simulink model "tqdtqr_rebuild_V3"  (R2021b)
settings: Solver=VariableStepAuto  StartTime=0.0  StopTime=10.0  RelTol=1e-3
undefined symbols (not defined in the file): ATQD_AfterTqMinGain_X_Deg, ATQD_APSCreepBaseTqD_X_kph, ATQD_APSCreepBaseTqD_Y_Deg, ATQD_APSCreepBaseTqR_X_kph, ATQD_APSCreepBaseTqR_Y_Deg, ATQD_APSCreepIterm_X_kph, ATQD_APSCreepIterm_Y_kph, ATQD_APSCreepPterm_X_kph, ATQD_APSCreepPterm_Y_kph, ATQD_APSDecReq_X_kph, ATQD_APSDecReq_Y_mps2, ATQD_APSDecReqCMD_X_kph, ATQD_APSDecReqTs_X_pct, ATQD_APSDecTimeGain_X_Deg, ATQD_APSDecTimeGain_Y_s, ATQD_APSReqLowSpd_X_Deg, ATQD_AutoHoldReleaseBPS_X_Deg, ATQD_AWDLoadTrqnsGain_X_kg, ATQD_AWDLoadTrqnsGain_Y_pct, ATQD_BOSEnBPSPosn_X_kph, ATQD_BOSMap_X_rpm, ATQD_BOSMap_Y_pct, ATQD_CreepBaseTqD_X_kph, ATQD_CreepBaseTqD_Y_Deg, ATQD_CreepBaseTqR_X_kph, ATQD_CreepBaseTqR_Y_Deg, ATQD_CreepBPSDisPosn_X_Deg, ATQD_CreepBPSDisPosnR_X_Deg, ATQD_CreepBPSEnPosn_X_Deg, ATQD_CreepBPSEnPosnR_X_Deg, ATQD_CreepDeltaTq_X_kph, ATQD_CreepIterm_X_kph, ATQD_CreepIterm_Y_kph, ATQD_CreepItermMaxLimit_X_pct, ATQD_CreepPreloadTime_X_kph, ATQD_CreepPreloadTq_X_kph, ATQD_CreepPreloadTq_Y_s, ATQD_CreepProtTq_X_Deg, ATQD_CreepPterm_X_kph, ATQD_CreepPterm_Y_kph, ATQD_CreepRrTqSpRat_X_rpm, ATQD_CreepRrTqSpRat_Y_Nm, ATQD_CreepTargetSpdD_X_pct, ATQD_CreepTargetSpdR_X_pct, ATQD_CreepUpLimitTq_X_rpm, ATQD_DecIneOPDHoldEnDelay_X_Deg, ATQD_DecIneOPDHoldEnDelay_Y_bar, ATQD_ECOTqMapD_X_rpm, ATQD_ECOTqMapD_Y_pct, ATQD_EMTqMapD_X_rpm, ATQD_EMTqMapD_Y_pct, ATQD_EOPDTqMapDCon_X_rpm, ATQD_EOPDTqMapDCon_Y_Deg, ATQD_EstInitVehWeight_X_c, ATQD_FAfterTqCMDGain_X_rpm, ATQD_FAfterTqCMDGain_Y_pct, ATQD_ForceLowSpd_X_Deg, ATQD_ForcePLimitSpd_X_Deg, ATQD_FrLossMAPLowV_X_rpm, ATQD_FrLossMAPLowV_Y_Nm ... (+949)
libraries: simulink x235, hcu_lib x208, tqr x63, tqd x6
(part 18 of 37)

== system tqdtqr_rebuild_V3/Input_Convert/Main function/DriverWhlTqDem function/PedalMapWhlTq ==
  note: Slide rate/SAS/YawRate regen torque
  note: According conditons use different torque, upper and lower limits
  note: Road slope
  note: Pedal map final torque
  note: Cancel ACC condition
  note: ACC shut off
  BSCPIn_outputs : Inport
  BSignalConvert_outputs : Inport  Port=2
  VTQD_PedAccTqEn_flg : Inport  Port=3
  VTQD_PedalTqCal_Nm : Inport  Port=4
  VTQD_PedalMapWhlTqMerge_Nm : Inport  Port=5
  BMain_outputs : Inport  Port=6
  BFunction_outputs : Inport  Port=7
  AND{,1..4,6} (6 alike) : Logic  AllPortsSameDT=off  OutDataTypeStr=boolean
  AND5 : Logic  Inputs=3  AllPortsSameDT=off  OutDataTypeStr=boolean
  AND7 : Logic  Operator=OR  AllPortsSameDT=off  OutDataTypeStr=boolean
  Abs{,1..3} (4 alike) : Abs
  Add : Sum  Inputs=+-
  Add1 : Sum
  Add13 : Sum  Inputs=+-
  Add2 : Sum
  Add3 : Sum
  Add4 : Sum  Inputs=+-
  Bus Selector : BusSelector  OutputSignals=VVMC_EstSlope_Deg,VINP_RrPTCSActive_flg,VINP_FrPTCSActive_flg,VINP_ADASACCSta_enum,VTQD_LowIdleAccPedal_flg,VVMC_ADASActive_flg,VVMC_ActMaxSlideRate_pct,VVMC_LongAcc_Gps,VINP_SASAngle_Deg,VINP_YawRate_degps,VVMC_ActStESCYaw_Dps,VINP_BrkPedalPos_pct,VTQD_ActAPSPosn_pct,VVMC_ADASWhlTqReq_Nm,VINP_HSAActive_flg
  Bus Selector1 : BusSelector  OutputSignals=VTQD_BrkSwSta_flg,VTQD_RollRegenDisable_flg,VTQD_TqTargetShaftSpd_rpm,VTQD_VehActSpd_kph
  Bus Selector2 : BusSelector  OutputSignals=VTQD_OPDHoldEnRel_flg
  Bus Selector3 : BusSelector  OutputSignals=VTQR_NoABSREDUWhlTqReq_Nm,VTQR_NoABSFEDUWhlTqReq_Nm
  Constant1 : Constant  Value=KTQD_RgnEnLatchSpd_kph
  Constant10 : Constant  Value=KTQD_ClimbMin_rpm
  Constant11 : Constant  Value=KTQD_PedalMapRDCUpLim_Nm
  Constant12 : Constant  Value=KTQD_PedalMapRDCLowLim_Nm
  Constant13 : Constant  Value=KTQD_GRADE_Deg_ovrdval
  Constant14 : Constant  Value=KTQD_PedalMapRDCUpLim_Nm
  Constant15 : Constant  Value=KTQD_TargetSlideRate_pct
  Constant16 : Constant  Value=KTQD_SlideRateDevUpLim_pct
  Constant17 : Constant  Value=KTQD_SlideRateDevLowLim_pct
  Constant18 : Constant  Value=KTQD_PedalMapRDCLowLim_Nm
  Constant19 : Constant  Value=KTQD_SlideRegEnLimitTq_Nm
  Constant20 : Constant  Value=KTQD_SlideRegEnLimitTq_Nm
  Constant21 : Constant  Value=KTQD_OrigPedTqLowLimSW_flg
  Constant22 : Constant  Value=KTQD_PedalMapRDCLowLim_Nm
  Constant23 : Constant  Value=KTQD_SlideRegenLowLim_Nm
  Constant24 : Constant  Value=KTQD_RgnEnLatchBrkPos_pct
  Constant25 : Constant  Value=ENUM_ADASACCSTA_SHUTOFF
  Constant26 : Constant  Value=KTQD_RgnEnLatchBrkPos_pct
  Constant27 : Constant  Value=KTQD_RgnEnLatchSlope_Deg
  Constant28 : Constant  Value=ZERO_FLOAT
  Constant29 : Constant  Value=ENUM_ADASACCSTA_STANDBY
  Constant30 : Constant  Value=ENUM_ADASACCSTA_OFF
  Constant31 : Constant  Value=KTQD_ACCOvrdCancelResPedTq_pct
  Constant32 : Constant  Value=KTQD_ACCOvrdCancelTqCtrl_flg
  Constant33 : Constant  Value=KVMC_ACCOvrdTestSW_flg
  Constant4 : Constant  Value=KTQD_GRADE_Deg_ovrdflg
  Constant5 : Constant  Value=KTQD_PedalMapClimbLowLim_Nm
  Constant69 : Constant  Value=KTQD_ACCOvrdCancelPedTqRat_Nm
  Constant72 : Constant  Value=ENUM_ADASACCSTA_OVERRIDE
  Delay : Delay  DelayLength=1
  Delay1 : Delay  DelayLength=1
  Delay2 : Delay  DelayLength=1
  Delay3 : Delay  DelayLength=1  InitialCondition=single(0)
      settings: AttributesFormatString=%<InitialCondition>
  Delay4 : Delay  DelayLength=1  InitialCondition=single(0)
      settings: AttributesFormatString=%<InitialCondition>
  Detect Decrease : simulink/Logic and Bit Operations/Detect Decrease  vinit=0.0  OutDataTypeStr=boolean
  Detect Increase : simulink/Logic and Bit Operations/Detect Increase  vinit=0.0  OutDataTypeStr=boolean
  Detect Increase1 : simulink/Logic and Bit Operations/Detect Increase  vinit=0.0  OutDataTypeStr=boolean
  Divide7 : Product  Inputs=**
  Equal : RelationalOperator  Operator===  OutDataTypeStr=boolean  RndMeth=Simplest
  Logical Operator2 : Logic  Operator=OR  Inputs=3  AllPortsSameDT=off  OutDataTypeStr=boolean
  Logical Operator3 : Logic  Operator=OR  AllPortsSameDT=off  OutDataTypeStr=boolean
  MTQD_OrigPedTqLowLim_Z_Nm : Lookup_n-D  BreakpointsForDimension1=ATQD_OrigPedTqLowLim_Y_pct  BreakpointsForDimension2=ATQD_OrigPedTqLowLim_X_Deg  Table=MTQD_OrigPedTqLowLim_Z_Nm  ExtrapMethod=Clip  InternalRulePriority=Speed  RndMeth=Simplest  InputSameDT=on
      settings: InputPortMap=u0,u1
  MTQD_PedalMapClimbUpLim_Z_Nm : Lookup_n-D  BreakpointsForDimension1=ATQD_PedalMapClimbUpLim_Y_Deg  BreakpointsForDimension2=ATQD_PedalMapClimbUpLim_X_rpm  Table=MTQD_PedalMapClimbUpLim_Z_Nm  ExtrapMethod=Clip  InternalRulePriority=Speed  RndMeth=Simplest  InputSameDT=on
      settings: InputPortMap=u0,u1
  "MTQD_SlideRegenTqGain_Z_Nm " : Lookup_n-D  BreakpointsForDimension1=ATQD_SlideRegenTqGain_Y_pct  BreakpointsForDimension2=ATQD_SlideRegenTqGain_X_Gps  Table=MTQD_SlideRegenTqGain_Z_Nm  ExtrapMethod=Clip  InternalRulePriority=Speed  RndMeth=Simplest  InputSameDT=on
      settings: InputPortMap=u0,u1
  MTQD_YawTqLowLim_Y_Nm : Lookup_n-D  NumberOfTableDimensions=1  BreakpointsForDimension1=ATQD_YawTqLowLim_X_degps  Table=MTQD_YawTqLowLim_Y_Nm  ExtrapMethod=Clip  InternalRulePriority=Speed  RndMeth=Simplest  InputSameDT=on
  Max{,1..3} (4 alike) : MinMax  Function=max  Inputs=2
  Min : MinMax  Inputs=2
  NOT : Logic  Operator=NOT  AllPortsSameDT=off  OutDataTypeStr=boolean
  NOT1 : Logic  Operator=NOT  AllPortsSameDT=off  OutDataTypeStr=boolean
  OR{,1..3} (4 alike) : Logic  Operator=OR  AllPortsSameDT=off  OutDataTypeStr=boolean
  Relational Operator{,1,3,6,9,12} (6 alike) : RelationalOperator  Operator=<=  OutDataTypeStr=boolean  RndMeth=Simplest
  Relational Operator10 : RelationalOperator  OutDataTypeStr=boolean  RndMeth=Simplest
  Relational Operator11 : RelationalOperator  OutDataTypeStr=boolean  RndMeth=Simplest
  Relational Operator2 : RelationalOperator  Operator=>  OutDataTypeStr=boolean  RndMeth=Simplest
  Relational Operator4 : RelationalOperator  Operator===  OutDataTypeStr=boolean  RndMeth=Simplest
  Relational Operator5 : RelationalOperator  Operator=>  OutDataTypeStr=boolean  RndMeth=Simplest
  Relational Operator7 : RelationalOperator  Operator===  OutDataTypeStr=boolean  RndMeth=Simplest
  Relational Operator8 : RelationalOperator  Operator===  OutDataTypeStr=boolean  RndMeth=Simplest
  SR_Latch{,1..4} (5 alike) : hcu_lib/Basic_Blocks/SR_Latch
  Saturation Dynamic{,1..4} (5 alike) : simulink/Discontinuities/Saturation Dynamic  OutMin=[]  OutMax=[]  OutDataTypeStr=Inherit: Same as second input  OutDataType=fixdt(1, 16)  OutScaling=2^-10  DoSatur=off
  Switch{3..8,10..12} (9 alike) : Switch  Criteria=u2 ~= 0
      Switch10 settings: AttributesFormatString=%<Criteria>
      Switch11 settings: AttributesFormatString=%<Criteria>
      Switch12 settings: AttributesFormatString=%<Criteria>
      Switch3 settings: AttributesFormatString=%<Criteria>
      Switch4 settings: AttributesFormatString=%<Criteria>
      Switch6 settings: AttributesFormatString=%<Criteria>
      Switch7 settings: AttributesFormatString=%<Criteria>
      Switch8 settings: AttributesFormatString=%<Criteria>
  Switch9 : Switch  Criteria=u2 > Threshold
  Triggered Subsystem : Subsystem  TreatAsAtomicUnit=on
  Unit Delay : UnitDelay  SampleTime=-1  HasFrameUpgradeWarning=on
  VTQD_PedalMapWhlTq_Nm : Outport
  VTQD_PreDecTqLowLim_Nm : Outport  Port=2
  VTQD_RegenTqLimitEn_flg : Outport  Port=3
  VTQD_SlideRegenLimTq_Nm : Outport  Port=4
  wires:
  [VTQD_RollRegenDisableReq_flg] -> Detect Decrease/1
  Relational Operator5/1 -> AND4/1
  [VTQR_NoABSFEDUWhlTqReq_Nm] -> Delay4/1
  [VTQD_BrkSwSta_flg] -> OR/2
  [VTQD_ACCCancelMemTq_Nm] -> Relational Operator11/2
  [VINP_BrkPedalPos_pct] -> Relational Operator5/1
  Constant5/1 -> Saturation Dynamic/3
  SR_Latch2/1 -> Switch9/2, Switch10/2  "VTQD_BrkRgnLatchEn_flg"
  [VTQD_LowIdleAccPedal_flg] -> NOT1/1
  Relational Operator3/1 -> AND7/1
  Switch9/1 -> [VTQD_BrkRgnLatchTqLim_Nm]  "VTQD_BrkRgnLatchTqLim_Nm"
  Delay1/1 -> OR1/1
  Constant24/1 -> Relational Operator3/2
  Constant69/1 -> Divide7/2
  [VTQD_ACCCancelMemTq_Nm] -> Max2/2
  Triggered Subsystem/2(Out2) -> [VTQD_ACCCancelMemPosn_pct]  "VTQD_ACCCancelMemPosn_pct"
  AND7/1 -> SR_Latch2/2
  Relational Operator10/1 -> Switch11/2
  Max2/1 -> Switch11/1
  AND5/1 -> SR_Latch4/1, Detect Increase1/1
  Relational Operator11/1 -> OR3/2
  Add3/1 -> Max3/2
  [VTQD_ActAPSPosn_pct] -> Relational Operator10/1
  Constant21/1 -> AND2/2
  Constant28/1 -> Min/2
  [VTQD_ACCCancelMemTq_Nm] -> Add3/1
  [VVMC_EstSlope_Deg] -> Switch5/3
  [VTQD_PedalTqCal_Nm] -> Switch12/1
  Min/1 -> Switch9/1
  [VVMC_EstSlope_Deg] -> Relational Operator6/1
  Relational Operator6/1 -> AND4/2
  [VINP_BrkPedalPos_pct] -> Relational Operator3/1
  Switch11/1 -> Switch7/1
  SR_Latch4/1 -> [VTQD_ACCCancelDet_flg]  "VTQD_ACCCancelDet_flg"
  OR2/1 -> AND5/2
  [VTQD_VehActSpd_kph] -> Relational Operator12/1
  Abs3/1 -> MTQD_OrigPedTqLowLim_Z_Nm/2
  Triggered Subsystem/1(Out1) -> [VTQD_ACCCancelMemTq_Nm]  "VTQD_ACCCancelMemTq_Nm"
  [VINP_YawRate_degps] -> Abs2/1
  Relational Operator9/1 -> OR3/1
  [VVMC_ActStESCYaw_degps] -> Add4/2
  Relational Operator8/1 -> OR2/2
  [VTQD_ActAPSPosn_pct] -> Add13/1
  AND2/1 -> Switch8/2
  [VVMC_LastADASWhlTqReq_Nm] -> Triggered Subsystem/1(in1)
  [VTQD_ActPedalMapWhlTq_Nm] -> Max3/1
  [VTQD_ActPedalMapWhlTq_Nm] -> Max2/1
  [VTQD_SlideTqLowLim_Nm] -> Switch9/3
  [VTQD_ActPedalMapWhlTq_Nm] -> Switch7/3
  [VTQD_OrigPedalMapWhlTq_Nm] -> Relational Operator2/1
  Switch4/1 -> [VTQD_ActPedalMapWhlTq_Nm]  "VTQD_ActPedalMapWhlTq_Nm"
  Constant16/1 -> Saturation Dynamic3/1
  Constant22/1 -> Saturation Dynamic4/1
  [VTQD_SlideRegenLimTq_Nm] -> Switch8/1
  Constant17/1 -> Saturation Dynamic3/3
  MTQD_PedalMapClimbUpLim_Z_Nm/1 -> Saturation Dynamic/1  "VTQD_PedalMapClimbUpLim_Nm"
  Max1/1 -> [VTQD_PreDecTqLowLim_Nm]  "VTQD_PreDecTqLowLim_Nm"
  Detect Increase/1 -> AND3/2
  Relational Operator1/1 -> AND1/2
  [VINP_ADASACCSta_enum] -> Unit Delay/1
  Detect Decrease/1 -> AND1/1
  Switch12/1 -> [VTQD_OrigPedalMapWhlTq_Nm]  "VTQD_OrigPedalMapWhlTq_Nm"
  Saturation Dynamic/1 -> Switch3/1
  [VINP_SASAngle_Deg] -> Abs3/1
  [VTQD_OrigPedTqLowLim_Nm] -> Saturation Dynamic2/3
  Delay/1 -> [VTQD_LastSlideRegenLimTq_Nm]  "VTQD_LastSlideRegenLimTq_Nm"
  [VTQD_ACCCancelMemPosn_pct] -> Relational Operator10/2
  Constant30/1 -> Relational Operator8/2
  [VTQD_PedAccTqEn_flg] -> Switch12/2
  [VTQD_OrigPedalMapWhlTq_Nm] -> Relational Operator1/1
  [VVMC_ADASActive_flg] -> Logical Operator2/3
  MTQD_OrigPedTqLowLim_Z_Nm/1 -> [VTQD_SlideTqLowLim_Nm], Max1/1  "VTQD_SlideTqLowLim_Nm"
  [VINP_ADASACCSta_enum] -> Relational Operator7/1
  [VTQD_PedalMapWhlTqMerge_Nm] -> Switch12/3
  Relational Operator4/1 -> AND5/1
  Constant33/1 -> AND6/2
  OR3/1 -> SR_Latch4/2
  Switch7/1 -> [VTQD_PedalMapWhlTq_Nm]  "VTQD_PedalMapWhlTq_Nm"
  Constant27/1 -> Relational Operator6/2
  Abs/1 -> Relational Operator/1
  [VVMC_ActMaxSlideRate_pct] -> MTQD_OrigPedTqLowLim_Z_Nm/1
  [VINP_FrPTCSActive_flg] -> Logical Operator3/2
  AND/1 -> Switch3/2  "VTQD_ActHSAActive_flg"
  Constant15/1 -> Add/2
  Constant26/1 -> Relational Operator5/2
  NOT/1 -> SR_Latch/2
  [VTQD_ADASShutOff_flg] -> Logical Operator2/1
  Divide7/1 -> Add3/2
  Detect Increase1/1 -> Triggered Subsystem/Trigger
  Constant72/1 -> Relational Operator4/2
  Relational Operator12/1 -> AND7/2
  [VTQD_ActAPSPosn_pct] -> Relational Operator9/1
  [VTQD_ActPedalMapWhlTq_Nm] -> Relational Operator11/1
  Logical Operator2/1 -> Switch4/2
  Add4/1 -> MTQD_YawTqLowLim_Y_Nm/1  "VTQD_TqLowLimYawDev_degps"
  Add13/1 -> Divide7/1
  [VTQR_NoABSREDUWhlTqReq_Nm] -> Delay3/1
  "MTQD_SlideRegenTqGain_Z_Nm "/1 -> Add1/1  "VTQD_SlideRegenLimTqGain_Nm"
  Constant29/1 -> Relational Operator7/2
  [VTQD_PreDecTqLowLim_Nm] -> Switch8/3
  [VTQD_ActAPSPosn_pct] -> Triggered Subsystem/2(In2)
  Switch6/1 -> Add1/2
  Constant4/1 -> Switch5/2
  Switch5/1 -> [VTQD_GRADE_Deg]  "VTQD_GRADE_Deg"
  Constant32/1 -> AND5/3
  Saturation Dynamic4/1 -> Delay/1, [VTQD_SlideRegenLimTq_Nm]  "VTQD_SlideRegenLimTq_Nm"
  Saturation Dynamic3/1 -> "MTQD_SlideRegenTqGain_Z_Nm "/1  "VTQD_SlideRateDev_pct"
  [VVMC_ActMaxSlideRate_pct] -> Add/1
  Constant23/1 -> Saturation Dynamic4/3
  SR_Latch1/1 -> [VTQD_RegenTqLimitEn_flg], Switch6/2  "VTQD_RegenTqLimitEn_flg"
  AND1/1 -> SR_Latch1/1
  Add/1 -> Saturation Dynamic3/2
  Relational Operator2/1 -> SR_Latch1/2
  Add1/1 -> Saturation Dynamic4/2
  [VVMC_LongAcc_Gps] -> "MTQD_SlideRegenTqGain_Z_Nm "/2
  Constant11/1 -> Saturation Dynamic1/1
  Saturation Dynamic2/1 -> Switch3/3
  [VTQD_TqTargetShaftSpd_rpm] -> Abs1/1
  SR_Latch/1 -> AND/1
  Constant13/1 -> Switch5/1
  Relational Operator/1 -> AND/2, NOT/1
  AND6/1 -> Switch7/2
  Switch3/1 -> Switch4/3
  Constant20/1 -> Relational Operator2/2
  MTQD_YawTqLowLim_Y_Nm/1 -> Max1/2  "VTQD_YawTqLowLim_Nm"
  [VTQD_OPDHoldEnRel_flg] -> Delay1/1
  OR1/1 -> SR_Latch/1
  Constant14/1 -> Saturation Dynamic2/1
  Constant19/1 -> Relational Operator1/2
  Constant1/1 -> Relational Operator12/2
  [VINP_HSAActive_flg] -> OR1/2
  [VINP_ADASACCSta_enum] -> Equal/1
  Add2/1 -> Switch10/3
  Delay2/1 -> Switch10/1
  Constant10/1 -> Relational Operator/2
  AND4/1 -> SR_Latch2/1
  Switch10/1 -> Min/1, Delay2/1
  [VTQD_RegenTqLimitEn_flg] -> AND2/1
  [VINP_ADASACCSta_enum] -> Relational Operator8/1
  Abs1/1 -> MTQD_PedalMapClimbUpLim_Z_Nm/2
  Abs2/1 -> Add4/1
  Constant18/1 -> Switch6/3
  Relational Operator7/1 -> OR2/1
  Constant31/1 -> Relational Operator9/2
  Saturation Dynamic1/1 -> Switch4/1
  OR/1 -> SR_Latch3/2
  Max/1 -> [VTQD_OrigPedTqLowLim_Nm]  "VTQD_OrigPedTqLowLim_Nm"
  [VTQD_BrkRgnLatchTqLim_Nm] -> Max/2
  [VTQD_GRADE_Deg] -> MTQD_PedalMapClimbUpLim_Z_Nm/1
  Constant12/1 -> Saturation Dynamic1/3
  [VINP_RrPTCSActive_flg] -> Logical Operator3/1
  Switch8/1 -> Max/1
  [VTQD_TqTargetShaftSpd_rpm] -> Abs/1
  [VTQD_ACCCancelMemPosn_pct] -> Add13/2
  [VTQD_LastSlideRegenLimTq_Nm] -> Switch6/1
  Unit Delay/1 -> Relational Operator4/1
  Logical Operator3/1 -> AND3/1
  SR_Latch3/1 -> [VTQD_ADASShutOff_flg]  "VTQD_ADASShutOff_flg"
  Equal/1 -> Detect Increase/1
  [VTQD_RollRegenDisableReq_flg] -> Logical Operator2/2
  Constant25/1 -> Equal/2
  Max3/1 -> Switch11/3
  AND3/1 -> SR_Latch3/1
  [VTQD_ACCCancelDet_flg] -> AND6/1
  NOT1/1 -> OR/1
  VTQD_PedAccTqEn_flg/1 -> [VTQD_PedAccTqEn_flg]
  VTQD_PedalTqCal_Nm/1 -> [VTQD_PedalTqCal_Nm]
  BSCPIn_outputs/1 -> Bus Selector/1
  BSignalConvert_outputs/1 -> Bus Selector1/1
  Bus Selector/1 -> [VVMC_EstSlope_Deg]  "<VVMC_EstSlope_Deg>"
  Bus Selector/2 -> [VINP_RrPTCSActive_flg]  "<VINP_RrPTCSActive_flg>"
  Bus Selector/3 -> [VINP_FrPTCSActive_flg]  "<VINP_FrPTCSActive_flg>"
  Bus Selector/4 -> [VINP_ADASACCSta_enum]  "<VINP_ADASACCSta_enum>"
  Bus Selector/5 -> [VTQD_LowIdleAccPedal_flg]  "<VTQD_LowIdleAccPedal_flg>"
  Bus Selector1/1 -> [VTQD_BrkSwSta_flg]  "<VTQD_BrkSwSta_flg>"
  Bus Selector1/2 -> [VTQD_RollRegenDisableReq_flg]  "<VTQD_RollRegenDisable_flg>"
  Bus Selector/6 -> [VVMC_ADASActive_flg]  "<VVMC_ADASActive_flg>"
  Bus Selector/7 -> [VVMC_ActMaxSlideRate_pct]  "<VVMC_ActMaxSlideRate_pct>"
  Bus Selector/8 -> [VVMC_LongAcc_Gps]  "<VVMC_LongAcc_Gps>"
  Bus Selector/9 -> [VINP_SASAngle_Deg]  "<VINP_SASAngle_Deg>"
  Bus Selector/10 -> [VINP_YawRate_degps]  "<VINP_YawRate_degps>"
  Bus Selector/11 -> [VVMC_ActStESCYaw_degps]  "<VVMC_ActStESCYaw_Dps>"
  Bus Selector/12 -> [VINP_BrkPedalPos_pct]  "<VINP_BrkPedalPos_pct>"
  Bus Selector/13 -> [VTQD_ActAPSPosn_pct]  "<VTQD_ActAPSPosn_pct>"
  Bus Selector/14 -> [VVMC_LastADASWhlTqReq_Nm]  "<VVMC_ADASWhlTqReq_Nm>"
  VTQD_PedalMapWhlTqMerge_Nm/1 -> [VTQD_PedalMapWhlTqMerge_Nm]
  Bus Selector1/3 -> [VTQD_TqTargetShaftSpd_rpm]  "<VTQD_TqTargetShaftSpd_rpm>"
  Bus Selector/15 -> [VINP_HSAActive_flg]  "<VINP_HSAActive_flg>"
  [VTQD_PedalMapWhlTq_Nm] -> VTQD_PedalMapWhlTq_Nm/1
  [VTQD_PreDecTqLowLim_Nm] -> VTQD_PreDecTqLowLim_Nm/1
  [VTQD_OrigPedalMapWhlTq_Nm] -> Saturation Dynamic1/2
  [VTQD_OrigPedalMapWhlTq_Nm] -> Saturation Dynamic/2
  [VTQD_OrigPedalMapWhlTq_Nm] -> Saturation Dynamic2/2
  [VTQD_RegenTqLimitEn_flg] -> VTQD_RegenTqLimitEn_flg/1
  [VTQD_SlideRegenLimTq_Nm] -> VTQD_SlideRegenLimTq_Nm/1
  Bus Selector1/4 -> [VTQD_VehActSpd_kph]  "<VTQD_VehActSpd_kph>"
  BFunction_outputs/1 -> Bus Selector2/1
  Bus Selector2/1 -> [VTQD_OPDHoldEnRel_flg]  "<VTQD_OPDHoldEnRel_flg>"
  BMain_outputs/1 -> Bus Selector3/1
  Bus Selector3/1 -> [VTQR_NoABSREDUWhlTqReq_Nm]  "<VTQR_NoABSREDUWhlTqReq_Nm>"
  Bus Selector3/2 -> [VTQR_NoABSFEDUWhlTqReq_Nm]  "<VTQR_NoABSFEDUWhlTqReq_Nm>"
  Delay3/1 -> Add2/1
  Delay4/1 -> Add2/2

== system tqdtqr_rebuild_V3/Input_Convert/Main function/DriverWhlTqDem function/Preload system ==
  note: New preload torque
  note: Enable preload flag
  note: Preload torque
  note: OPD hold preload conditions
  note: ADAS preload conditions
  note: Shift preload conditions
  BSCPIn_outputs : Inport
  BSignalConvert_outputs : Inport  Port=2
  BFunction_outputs : Inport  Port=3
  VTQD_CreepEnable_flg : Inport  Port=4
  AND : Logic  Inputs=3  AllPortsSameDT=off  OutDataTypeStr=boolean
  AND{1..3,7..9,11} (7 alike) : Logic  AllPortsSameDT=off  OutDataTypeStr=boolean
  AND4 : Logic  Inputs=6  AllPortsSameDT=off  OutDataTypeStr=boolean
  AND5 : Logic  Inputs=4  AllPortsSameDT=off  OutDataTypeStr=boolean
  Abs{,1..4} (5 alike) : Abs
  Bus Selector : BusSelector  OutputSignals=VVMC_ACCVehHoldReq_flg,task_time_s,VINP_VehSpeed_kph,VVMC_ADASActive_flg,VTQD_LowIdleAccPedal_flg,VINP_FrEDURealTMTq_Nm,VINP_RrEDURealTMTq_Nm,VDDM_VehMalfunLevel_enum,VVMC_APSActive_flg
  Bus Selector1 : BusSelector  OutputSignals=VTQD_FrShaftSpd_rpm,VTQD_RrShaftSpd_rpm,VTQD_TqTargetShaftSpd_rpm,VTQD_VehActSpd_kph
  Bus Selector2 : BusSelector  OutputSignals=VTQD_GearActualPosn_enum,VTQD_APSReqTimer_s
  Constant1 : Constant  Value=KTQD_RrPreLoadBoundary_Nm
  Constant11 : Constant  Value=KTQD_ADASHoldPreLoadspd_kph
  Constant12 : Constant  Value=KTQD_ADASHoldDelayEnTime_s
  Constant16 : Constant  Value=KTQD_PreLoadTqHold_rpm
  Constant17 : Constant  Value=ZERO_FLOAT
  Constant18 : Constant  Value=KTQD_OPDHoldPreLoadTime_s
  Constant19 : Constant  Value=KTQD_PreLoad_Holdtime_s
  Constant20 : Constant  Value=KTQD_APSZeroSpd_kph
  Constant21 : Constant  Value=ENUM_GEARACTUALPOSN_D
  Constant22 : Constant  Value=ENUM_GEARACTUALPOSN_D
  Constant{4,6,23..24} (4 alike) : Constant  Value=ENUM_GEARACTUALPOSN_R
  Constant27 : Constant  Value=KTQD_OPDHoldPreLoadBound_Nm
  Constant28 : Constant  Value=KTQD_OPDHoldPreLoadBound_Nm
  Constant29 : Constant  Value=KTQD_PreLoadDisSpd_kph
  Constant3 : Constant  Value=KTQD_RrPreLoadBoundary_Nm
  Constant42 : Constant  Value=KTQD_APSPreLoadHoldtime_s
  Constant45 : Constant  Value=ENUM_VEHMALFUNLEVEL_LEVEL3
  Constant5 : Constant  Value=ENUM_GEARACTUALPOSN_N
  Constant7 : Constant  Value=ENUM_GEARACTUALPOSN_P
  Constant9 : Constant  Value=KTQD_PreLoadTq_Nm
  Constant96 : Constant  Value=KTQD_FailsafeActiveSW_flg
  Delay : Delay  DelayLength=1  InitialCondition=boolean(0)
      settings: AttributesFormatString=%<InitialCondition>
  Delay1 : Delay  DelayLength=1
  Delay2 : Delay  DelayLength=1
  DelayEnable : hcu_lib/Basic_Blocks/DelayEnable
  Detect Increase : simulink/Logic and Bit Operations/Detect Increase  vinit=0.0  OutDataTypeStr=boolean
  Detect Increase1 : simulink/Logic and Bit Operations/Detect Increase  vinit=0.0  OutDataTypeStr=boolean
  Detect Increase2 : simulink/Logic and Bit Operations/Detect Increase  vinit=0.0  OutDataTypeStr=boolean
  Equal{1..4,6,8} (6 alike) : RelationalOperator  Operator===  OutDataTypeStr=boolean  RndMeth=Simplest
  Equal5 : RelationalOperator  Operator=~=  OutDataTypeStr=boolean  RndMeth=Simplest
  Equal7 : RelationalOperator  Operator=~=  OutDataTypeStr=boolean  RndMeth=Simplest
  GreaterThan : RelationalOperator  OutDataTypeStr=boolean  RndMeth=Simplest
  Logical Operator13 : Logic  AllPortsSameDT=off  OutDataTypeStr=boolean
  MTQD_PreLoadTq_Y_Nm : Lookup_n-D  NumberOfTableDimensions=1  BreakpointsForDimension1=ATQD_PreLoadTq_X_s  Table=MTQD_PreLoadTq_Y_Nm  ExtrapMethod=Clip  InternalRulePriority=Speed  RndMeth=Simplest  InputSameDT=on
  NOT{2..9} (8 alike) : Logic  Operator=NOT  AllPortsSameDT=off  OutDataTypeStr=boolean
  New Preload Torque : Subsystem
  OR14 : Logic  Operator=OR  Inputs=3  AllPortsSameDT=off  OutDataTypeStr=boolean
  OR3 : Logic  Operator=OR  Inputs=4  AllPortsSameDT=off  OutDataTypeStr=boolean
  OR{4..8} (5 alike) : Logic  Operator=OR  AllPortsSameDT=off  OutDataTypeStr=boolean
  Relational Operator{1..2,11..14} (6 alike) : RelationalOperator  Operator=<=  OutDataTypeStr=boolean  RndMeth=Simplest
  Relational Operator23 : RelationalOperator  OutDataTypeStr=boolean  RndMeth=Simplest
  Relational Operator3 : RelationalOperator  Operator=<  OutDataTypeStr=boolean  RndMeth=Simplest
  Relational Operator4 : RelationalOperator  Operator=>  OutDataTypeStr=boolean  RndMeth=Simplest
  Relational Operator5 : RelationalOperator  Operator=>  OutDataTypeStr=boolean  RndMeth=Simplest
  SR_Latch{1..6} (6 alike) : hcu_lib/Basic_Blocks/SR_Latch
  Switch5 : Switch  Criteria=u2 ~= 0
      settings: AttributesFormatString=%<Criteria>
  Switch6 : Switch  Criteria=u2 ~= 0
      settings: AttributesFormatString=%<Criteria>
  Switch8 : Switch  Criteria=u2 ~= 0
      settings: AttributesFormatString=%<Criteria>
  Timer1 : hcu_lib/Basic_Blocks/Timer
  Unit Delay{1..3,5} (4 alike) : UnitDelay  SampleTime=-1  HasFrameUpgradeWarning=on
  Unit Delay4 : UnitDelay  InitialCondition=boolean(0)  SampleTime=-1  HasFrameUpgradeWarning=on
      settings: AttributesFormatString=%<InitialCondition>
  Unit Delay6 : UnitDelay  InitialCondition=boolean(0)  SampleTime=-1  HasFrameUpgradeWarning=on
      settings: AttributesFormatString=%<InitialCondition>
  VTQD_PreLoadHold_flg : Outport
  VTQD_PreLoadPreEn_flg : Outport  Port=2
  VTQD_PreloadTq_Nm : Outport  Port=3
  VTQD_FrPreloadTq_Nm : Outport  Port=4
  VTQD_RrPreloadTq_Nm : Outport  Port=5
  wires:
  Equal8/1 -> AND9/2
  Unit Delay5/1 -> Equal3/1
  [VTQD_GearActualPosn_enum] -> Unit Delay3/1
  Equal7/1 -> AND9/1
  OR3/1 -> [VTQD_ShiftPreload_flg]  "VTQD_ShiftPreload_flg"
  Equal6/1 -> AND8/2
  Constant22/1 -> Equal6/2
  AND9/1 -> OR3/2
  Constant23/1 -> Equal7/2
  Equal2/1 -> AND1/2
  [VTQD_GearActualPosn_enum] -> Equal8/1
  Equal5/1 -> AND8/1
  Constant7/1 -> Equal4/2
  Unit Delay2/1 -> Equal5/1
  [VTQD_GearActualPosn_enum] -> Unit Delay1/1
  Equal4/1 -> AND2/2
  [VTQD_GearActualPosn_enum] -> Equal6/1
  [VTQD_GearActualPosn_enum] -> Unit Delay5/1
  AND2/1 -> OR3/4
  AND8/1 -> OR3/1
  Equal3/1 -> AND2/1
  [VTQD_GearActualPosn_enum] -> Equal4/1
  Constant6/1 -> Equal3/2
  Constant24/1 -> Equal8/2
  Unit Delay3/1 -> Equal7/1
  Constant4/1 -> Equal1/2
  Constant21/1 -> Equal5/2
  [VTQD_GearActualPosn_enum] -> Equal2/1
  Unit Delay1/1 -> Equal1/1
  Constant5/1 -> Equal2/2
  [VTQD_GearActualPosn_enum] -> Unit Delay2/1
  Equal1/1 -> AND1/1
  AND1/1 -> OR3/3
  Abs3/1 -> Relational Operator12/1
  SR_Latch5/1 -> AND4/1
  Delay/1 -> SR_Latch3/1
  AND4/1 -> [VTQD_OPDHoldPreLoadEn_flg]  "VTQD_OPDHoldPreLoadEn_flg"
  [VINP_ACCVehHoldReq_flg] -> AND7/2
  DelayEnable/1 -> AND5/1
  NOT8/1 -> OR6/1
  Detect Increase/1 -> SR_Latch3/2
  SR_Latch3/1 -> NOT5/1
  Relational Operator12/1 -> AND4/6
  [VINP_ACCVehHoldReq_flg] -> Detect Increase/1
  Relational Operator11/1 -> AND4/3
  [VTQD_HoldtimeEnd_flg] -> Delay1/1
  [VTQD_LowIdleAccPedal_flg] -> AND4/4
  NOT7/1 -> AND4/2
  Relational Operator13/1 -> AND4/5
  AND7/1 -> DelayEnable/1  "VTQD_ADASPreLoadHold_flg"
  Constant28/1 -> Relational Operator13/2
  Abs4/1 -> Relational Operator13/1
  Constant27/1 -> Relational Operator12/2
  Delay1/1 -> Detect Increase2/1
  SR_Latch6/1 -> OR6/2  "VTQD_PreLoadHoldtimeEnd_flg"
  [VTQD_LowIdleAccPedal_flg] -> NOT9/1
  NOT9/1 -> SR_Latch6/2
  Detect Increase2/1 -> SR_Latch6/1
  [VTQD_CreepEnable_flg] -> Delay2/1
  Delay2/1 -> NOT7/1
  Constant20/1 -> Relational Operator11/2
  [VINP_FrEDURealTMTq_Nm] -> Abs4/1
  [VINP_VehSpeed_kph] -> Relational Operator11/1
  Constant18/1 -> Relational Operator5/2
  Relational Operator5/1 -> Detect Increase1/1, NOT8/1
  Detect Increase1/1 -> SR_Latch5/1
  [VTQD_APSReqTimer_s] -> Relational Operator5/1
  [VTQD_LowIdleAccPedal_flg] -> AND5/4
  NOT5/1 -> AND7/1
  [VVMC_ADASActive_flg] -> AND5/3
  Constant12/1 -> DelayEnable/2
  Constant11/1 -> Relational Operator3/2
  Relational Operator3/1 -> AND5/2
  OR6/1 -> SR_Latch5/2
  AND5/1 -> [VTQD_ADASPreLoadEn_flg]  "VTQD_ADASPreLoadEn_flg"
  [VINP_VehSpeed_kph] -> Relational Operator3/1
  [VINP_RrEDURealTMTq_Nm] -> Abs3/1
  [VTQD_HoldtimeEnd_flg] -> Delay/1
  [task_time_s] -> DelayEnable/3  "task_time_s"
  AND/1 -> SR_Latch2/1
  AND11/1 -> OR8/2
  [VTQD_HoldtimeEnd_flg] -> Unit Delay6/1
  Relational Operator14/1 -> AND11/2
  Constant45/1 -> Relational Operator23/2
  Unit Delay4/1 -> OR4/1
  [VTQD_PreLoadHold_flg] -> AND11/1
  NOT4/1 -> OR14/2
  Constant29/1 -> Relational Operator14/2
  [VDDM_VehMalfunLevel_enum] -> Relational Operator23/1
  OR14/1 -> SR_Latch2/2
  Constant3/1 -> Relational Operator2/2
  [VVMC_APSActive_flg] -> Switch8/2
  Switch8/1 -> GreaterThan/2, Timer1/4
  OR5/1 -> [VTQD_PreLoadPreEn_flg], AND/3  "VTQD_PreLoadPreEn_flg"
  [VTQD_ShiftPreload_flg] -> OR7/2
  [task_time_s] -> Timer1/3
  [VTQD_HoldtimeEnd_flg] -> Unit Delay4/1
  Logical Operator13/1 -> OR14/3
  Unit Delay6/1 -> OR14/1
  Timer1/1 -> [VTQD_PreLoadHoldtime_s], GreaterThan/1  "VTQD_PreLoadHoldtime_s"
  Relational Operator1/1 -> AND/2
  [VTQD_OPDHoldPreLoadEn_flg] -> OR7/1
  GreaterThan/1 -> OR8/1
  Constant19/1 -> Switch8/3
  SR_Latch2/1 -> [VTQD_PreLoadHold_flg], NOT2/1, Timer1/1  "VTQD_PreLoadHold_flg"
  OR8/1 -> [VTQD_HoldtimeEnd_flg]  "VTQD_HoldtimeEnd_flg"
  NOT2/1 -> Timer1/2
  [VINP_FrEDURealTMTq_Nm] -> Abs1/1
  [VTQD_LowIdleAccPedal_flg] -> NOT4/1
  SR_Latch1/1 -> OR5/1
  NOT3/1 -> OR4/2
  Constant1/1 -> Relational Operator1/2
  Constant96/1 -> Logical Operator13/2
  [VTQD_VehActSpd_kph] -> Relational Operator14/1
  Abs1/1 -> Relational Operator2/1
  Constant42/1 -> Switch8/1
  Abs/1 -> Relational Operator1/1
  Relational Operator23/1 -> Logical Operator13/1
  [VINP_RrEDURealTMTq_Nm] -> Abs/1
  OR7/1 -> SR_Latch1/1
  [VTQD_ADASPreLoadEn_flg] -> OR5/2
  [VTQD_LowIdleAccPedal_flg] -> NOT3/1
  OR4/1 -> SR_Latch1/2
  Relational Operator2/1 -> AND/1
  BFunction_outputs/1 -> Bus Selector2/1
  BSignalConvert_outputs/1 -> Bus Selector1/1
  BSCPIn_outputs/1 -> Bus Selector/1
  [VTQD_PreLoadHold_flg] -> New Preload Torque/1(VTQD_PreLoadHold_flg)
  New Preload Torque/1(VTQD_FrPreloadTq_Nm) -> [VTQD_FrPreloadTq_Nm]
  [VTQD_RrShaftSpd_rpm] -> New Preload Torque/4(VTQD_RrShaftSpd_rpm)
  New Preload Torque/2(VTQD_RrPreloadTq_Nm) -> [VTQD_RrPreloadTq_Nm]
  [VTQD_PreLoadHoldtime_s] -> New Preload Torque/2(VTQD_PreLoadHoldtime_s)
  [VTQD_FrShaftSpd_rpm] -> New Preload Torque/3(VTQD_FrShaftSpd_rpm)
  Bus Selector2/1 -> [VTQD_GearActualPosn_enum]  "<VTQD_GearActualPosn_enum>"
  Bus Selector/1 -> [VINP_ACCVehHoldReq_flg]  "<VVMC_ACCVehHoldReq_flg>"
  Bus Selector/2 -> [task_time_s]  "<task_time_s>"
  Bus Selector/3 -> [VINP_VehSpeed_kph]  "<VINP_VehSpeed_kph>"
  Bus Selector/4 -> [VVMC_ADASActive_flg]  "<VVMC_ADASActive_flg>"
  Bus Selector/5 -> [VTQD_LowIdleAccPedal_flg]  "<VTQD_LowIdleAccPedal_flg>"
  Bus Selector/6 -> [VINP_FrEDURealTMTq_Nm]  "<VINP_FrEDURealTMTq_Nm>"
  Bus Selector/7 -> [VINP_RrEDURealTMTq_Nm]  "<VINP_RrEDURealTMTq_Nm>"
  Bus Selector/8 -> [VDDM_VehMalfunLevel_enum]  "<VDDM_VehMalfunLevel_enum>"
  Bus Selector/9 -> [VVMC_APSActive_flg]  "<VVMC_APSActive_flg>"
  Bus Selector1/1 -> [VTQD_FrShaftSpd_rpm]  "<VTQD_FrShaftSpd_rpm>"
  Bus Selector1/2 -> [VTQD_RrShaftSpd_rpm]  "<VTQD_RrShaftSpd_rpm>"
  [VTQD_PreLoadPreEn_flg] -> VTQD_PreLoadPreEn_flg/1
  [VTQD_PreLoadHold_flg] -> VTQD_PreLoadHold_flg/1
  Relational Operator4/1 -> AND3/2
  NOT6/1 -> SR_Latch4/2
  [VTQD_TqTargetShaftSpd_rpm] -> Abs2/1
  [VTQD_PreLoadHold_flg] -> AND3/1
  Constant17/1 -> Switch6/1
  MTQD_PreLoadTq_Y_Nm/1 -> Switch6/3
  [VTQD_PreLoadHoldtime_s] -> MTQD_PreLoadTq_Y_Nm/1
  Constant16/1 -> Relational Operator4/2
  SR_Latch4/1 -> Switch6/2
  [VTQD_PreLoadHold_flg] -> NOT6/1
  AND3/1 -> SR_Latch4/1
  Abs2/1 -> Relational Operator4/1
  [VTQD_PreloadTq_Nm] -> VTQD_PreloadTq_Nm/1
  Bus Selector1/3 -> [VTQD_TqTargetShaftSpd_rpm]  "<VTQD_TqTargetShaftSpd_rpm>"
  VTQD_CreepEnable_flg/1 -> [VTQD_CreepEnable_flg]
  [VTQD_RrPreloadTq_Nm] -> VTQD_RrPreloadTq_Nm/1
  [VTQD_FrPreloadTq_Nm] -> VTQD_FrPreloadTq_Nm/1
  Bus Selector1/4 -> [VTQD_VehActSpd_kph]  "<VTQD_VehActSpd_kph>"
  [VVMC_APSActive_flg] -> Switch5/2
  Constant9/1 -> Switch5/1
  Switch5/1 -> [VTQD_PreloadTq_Nm]  "VTQD_PreloadTq_Nm"
  Switch6/1 -> Switch5/3
  Bus Selector2/2 -> [VTQD_APSReqTimer_s]  "<VTQD_APSReqTimer_s>"

== system tqdtqr_rebuild_V3/Input_Convert/Main function/DriverWhlTqDem function/Rock Mode torque  ==
  note: Escape mode conditions
  note: Check wheels skip
  note: Calculate escape mode Tq
  note: Rock mode TCS flag
  note: Rock mode enable flag from IVI
  BSCPIn_outputs : Inport
  BSignalConvert_outputs : Inport  Port=2
  BFunction_outputs : Inport  Port=3
  VTQR_FShaftSpdTqLimLow_flg : Inport  Port=4
  VTQR_FTimerTqLimLow_flg : Inport  Port=5
  VTQR_RShaftSpdTqLimLow_flg : Inport  Port=6
  VTQR_RTimerTqLimLow_flg : Inport  Port=7
  AND{1..2,6,10,12..13,17} (7 alike) : Logic  AllPortsSameDT=off  OutDataTypeStr=boolean
  AND11 : Logic  Inputs=3  AllPortsSameDT=off  OutDataTypeStr=boolean
  AND14 : Logic  Inputs=3  AllPortsSameDT=off  OutDataTypeStr=boolean
  Abs{5..9} (5 alike) : Abs
  Add{,1..3} (4 alike) : Sum  Inputs=+-
  Bus Selector : BusSelector  OutputSignals=task_time_s,VTQD_ActAPSPosn_pct,VINP_LFRawWhlSpeed_kph,VINP_LRRawWhlSpeed_kph,VINP_RFRawWhlSpeed_kph,VINP_RRRawWhlSpeed_kph,VVMC_LongAcc_Gps,VINP_IVIEscapeModeCmd_flg,VPMM_SysPowerMode_enum,VINP_ESCOFFStatus_enum,VINP_FrPTCSActive_flg,VINP_RrPTCSActive_flg
  Bus Selector1 : BusSelector  OutputSignals=VTQD_FrShaftSpd_rpm,VTQD_RrShaftSpd_rpm,VTQD_VehActSpd_kph
  Bus Selector2 : BusSelector  OutputSignals=VTQD_GearActualPosn_enum,VTQD_ActWhlSkipSta_enum
  Constant{1..3,30} (4 alike) : Constant  Value=KTQD_RocModeWhlSpdDely_cnt
  Constant119 : Constant  Value=KTQD_RockModeEnTime_s
  Constant120 : Constant  Value=ENUM_GEARACTUALPOSN_P
  Constant121 : Constant  Value=KTQD_RockModeEnSpd_kph
  Constant{122..125} (4 alike) : Constant  Value=ENUM_ESCOFFSTATUS_TCSANDESCOFF
  Constant127 : Constant  Value=ENUM_PWRSTASW_READY
  Constant128 : Constant  Value=ENUM_PWRSTASW_READY
  Constant129 : Constant  Value=KTQD_RockModeTCSReqHold_s
  Constant{4..6,31} (4 alike) : Constant  Value=KTQD_RocModeTqLimSpdDev_kph
  Constant38 : Constant  Value=KTQD_RocModeTqLimAccCon_Gps
  Constant43 : Constant  Value=KTQD_RockModeWhlSkipSta_enum
  Delay10 : Delay  DelayLength=1  InitialCondition=boolean(0)
      settings: AttributesFormatString=%<InitialCondition>
  Delay11 : Delay  DelayLength=1  InitialCondition=uint8(0)
      settings: AttributesFormatString=%<InitialCondition>
  Delay12 : Delay  DelayLength=1  InitialCondition=boolean(0)
      settings: AttributesFormatString=%<InitialCondition>
  Delay13 : Delay  DelayLength=1  InitialCondition=single(0)
      settings: AttributesFormatString=%<InitialCondition>
  Delay14 : Delay  DelayLength=1  InitialCondition=single(0)
      settings: AttributesFormatString=%<InitialCondition>
  Delay15 : Delay  DelayLength=1  InitialCondition=single(0)
      settings: AttributesFormatString=%<InitialCondition>
  Delay16 : Delay  DelayLength=1  InitialCondition=uint8(0)
      settings: AttributesFormatString=%<InitialCondition>
  Delay{3..6} (4 alike) : Delay  DelayLengthSource=Input port
      settings: InputPortMap=u0,p1
  Delay7 : Delay  Description=%<InitialCondition>  DelayLength=1  InitialCondition=boolean(0)
      settings: AttributesFormatString=%<InitialCondition>
  Delay9 : Delay  DelayLength=1  InitialCondition=boolean(0)
      settings: AttributesFormatString=%<InitialCondition>
  DelayEnable1 : hcu_lib/Basic_Blocks/DelayEnable
  DelayEnable2 : hcu_lib/Basic_Blocks/DelayEnable
  Detect Change : simulink/Logic and Bit Operations/Detect Change  vinit=0  OutDataTypeStr=boolean
  Detect Decrease : simulink/Logic and Bit Operations/Detect Decrease  vinit=0.0  OutDataTypeStr=boolean
  Detect Decrease1 : simulink/Logic and Bit Operations/Detect Decrease  vinit=boolean(0)  OutDataTypeStr=boolean
  Detect Decrease2 : simulink/Logic and Bit Operations/Detect Decrease  vinit=boolean(0)  OutDataTypeStr=boolean
  Detect Decrease3 : simulink/Logic and Bit Operations/Detect Decrease  vinit=boolean(0)  OutDataTypeStr=boolean
  Detect Increase{1..5} (5 alike) : simulink/Logic and Bit Operations/Detect Increase  vinit=boolean(0)  OutDataTypeStr=boolean
  Equal49 : RelationalOperator  Operator===  OutDataTypeStr=boolean  RndMeth=Simplest
  Equal50 : RelationalOperator  Operator===  OutDataTypeStr=boolean  RndMeth=Simplest
  Equal51 : RelationalOperator  Operator=~=  OutDataTypeStr=boolean  RndMeth=Simplest
  Equal52 : RelationalOperator  Operator=~=  OutDataTypeStr=boolean  RndMeth=Simplest
  Equal53 : RelationalOperator  Operator===  OutDataTypeStr=boolean  RndMeth=Simplest
  Hold : hcu_lib/Basic_Blocks/Hold  SystemSampleTime=-1  VariantActivationTime=update diagram  Latency=0  AutoFrameSizeCalculation=off
  MTQD_RockModeDisTime_Y_s : Lookup_n-D  NumberOfTableDimensions=1  BreakpointsForDimension1=ATQD_RockModeDisTime_X_rpm  Table=MTQD_RockModeDisTime_Y_s  InternalRulePriority=Speed  RndMeth=Simplest  InputSameDT=on
  MTQD_RockModePedTq_Z_Nm : Lookup_n-D  BreakpointsForDimension1=ATQD_RockModePedTq_Y_rpm  BreakpointsForDimension2=ATQD_RockModePedTq_X_pct  Table=MTQD_RockModePedTq_Z_Nm  InternalRulePriority=Speed  RndMeth=Simplest  InputSameDT=on
      settings: InputPortMap=u0,u1
  Max : MinMax  Function=max  Inputs=2
  Max2 : MinMax  Function=max  Inputs=2
  NOT10 : Logic  Operator=NOT  AllPortsSameDT=off  OutDataTypeStr=boolean
  NOT2 : Logic  Operator=NOT  AllPortsSameDT=off  OutDataTypeStr=boolean
  OR{5,8,10,12} (4 alike) : Logic  Operator=OR  AllPortsSameDT=off  OutDataTypeStr=boolean
  OR11 : Logic  Operator=OR  Inputs=4  AllPortsSameDT=off  OutDataTypeStr=boolean
  OR4 : Logic  Operator=OR  Inputs=6  AllPortsSameDT=off  OutDataTypeStr=boolean
  OR9 : Logic  Operator=OR  Inputs=4  AllPortsSameDT=off  OutDataTypeStr=boolean
  Relational Operator10 : RelationalOperator  Operator=~=  OutDataTypeStr=boolean  RndMeth=Simplest
  Relational Operator{15..18} (4 alike) : RelationalOperator  OutDataTypeStr=boolean  RndMeth=Simplest
  Relational Operator19 : RelationalOperator  Operator=<=  OutDataTypeStr=boolean  RndMeth=Simplest
  Relational Operator2 : RelationalOperator  Operator=<=  OutDataTypeStr=boolean  RndMeth=Simplest
  Relational Operator22 : RelationalOperator  Operator=>  OutDataTypeStr=boolean  RndMeth=Simplest
  Relational Operator9 : RelationalOperator  Operator===  OutDataTypeStr=boolean  RndMeth=Simplest
  SR_Latch1 : hcu_lib/Basic_Blocks/SR_Latch
  SR_Latch5 : hcu_lib/Basic_Blocks/SR_Latch
  SR_Latch7 : hcu_lib/Basic_Blocks/SR_Latch
  Switch24 : Switch  Criteria=u2 ~= 0
      settings: AttributesFormatString=%<Criteria>
  VTQD_IVIRockModeEn_flg : Outport
  VTQD_RockModeTCSReq_flg : Outport  Port=2
  VTQD_RockModePedTq_Nm : Outport  Port=3
  VTQD_RockModeTqLim_flg : Outport  Port=4
  wires:
  [VTQD_ActAPSPosn_pct] -> MTQD_RockModePedTq_Z_Nm/2
  [VTQD_RrShaftSpd_rpm] -> Max/2
  Max/1 -> MTQD_RockModePedTq_Z_Nm/1  "VTQD_MaxShaftSpd_rpm"
  MTQD_RockModePedTq_Z_Nm/1 -> [VTQD_RockModePedTq_Nm]  "VTQD_RockModePedTq_Nm"
  [VTQD_FrShaftSpd_rpm] -> Max/1
  [VINP_RRRawWhlSpeed_kph] -> Add3/1
  Relational Operator19/1 -> AND13/2
  Constant5/1 -> Relational Operator17/2
  [VTQD_WhlQuickSkip_flg] -> AND13/1
  Delay6/1 -> Add3/2
  Constant38/1 -> Relational Operator19/2
  AND13/1 -> [VTQD_WhlSpdQuickSkip_flg]  "VTQD_WhlSpdQuickSkip_flg"
  Abs7/1 -> Relational Operator17/1
  Delay5/1 -> Add2/2
  Abs5/1 -> Relational Operator15/1
  Delay3/1 -> Add/2
  Constant30/1 -> Delay3/2
  [VINP_RFRawWhlSpeed_kph] -> Add2/1
  [VINP_LRRawWhlSpeed_kph] -> Delay4/1
  [VINP_LRRawWhlSpeed_kph] -> Add1/1
  Constant4/1 -> Relational Operator15/2
  Add1/1 -> Abs6/1
  Delay4/1 -> Add1/2
  [VINP_RRRawWhlSpeed_kph] -> Delay6/1
  OR11/1 -> [VTQD_WhlQuickSkip_flg]  "VTQD_WhlQuickSkip_flg"
  [VINP_RFRawWhlSpeed_kph] -> Delay5/1
  Relational Operator17/1 -> OR11/3
  Relational Operator16/1 -> OR11/2
  Constant2/1 -> Delay5/2
  Constant3/1 -> Delay6/2
  Constant1/1 -> Delay4/2
  Abs6/1 -> Relational Operator16/1
  Constant31/1 -> Relational Operator16/2
  Relational Operator18/1 -> OR11/4
  [VVMC_LongAcc_Gps] -> Abs9/1
  [VINP_LFRawWhlSpeed_kph] -> Add/1
  Add2/1 -> Abs7/1
  Abs9/1 -> Relational Operator19/1
  Add3/1 -> Abs8/1
  Add/1 -> Abs5/1
  Abs8/1 -> Relational Operator18/1
  Relational Operator15/1 -> OR11/1
  [VINP_LFRawWhlSpeed_kph] -> Delay3/1
  Constant6/1 -> Relational Operator18/2
  OR9/1 -> AND12/1
  [VTQR_RShaftSpdTqLimLow_flg] -> OR9/1
  OR10/1 -> SR_Latch7/2
  AND12/1 -> Detect Decrease/1
  [VTQD_GearActualPosn_enum] -> Detect Change/1
  [VTQD_WhlSpdQuickSkip_flg] -> OR12/2
  AND17/1 -> [VTQD_RockModeTqLim_flg]  "VTQD_RockModeTqLim_flg"
  [VTQR_RTimerTqLimLow_flg] -> OR9/2
  Relational Operator22/1 -> AND17/1
  SR_Latch7/1 -> AND17/2
  [VTQD_ActWhlSkipSta_enum] -> Relational Operator22/1
  NOT10/1 -> OR10/1
  [VTQD_IVIRockModeEn_flg] -> NOT10/1
  Detect Decrease/1 -> OR12/1
  [VTQD_IVIRockModeEn_flg] -> AND12/2
  Constant43/1 -> Relational Operator22/2
  [VTQR_FShaftSpdTqLimLow_flg] -> OR9/3
  [VTQR_FTimerTqLimLow_flg] -> OR9/4
  OR12/1 -> SR_Latch7/1
  Detect Change/1 -> OR10/2
  BSCPIn_outputs/1 -> Bus Selector/1
  BSignalConvert_outputs/1 -> Bus Selector1/1
  BFunction_outputs/1 -> Bus Selector2/1
  Bus Selector1/1 -> [VTQD_FrShaftSpd_rpm]  "<VTQD_FrShaftSpd_rpm>"
  Bus Selector1/2 -> [VTQD_RrShaftSpd_rpm]  "<VTQD_RrShaftSpd_rpm>"
  Bus Selector/2 -> [VTQD_ActAPSPosn_pct]  "<VTQD_ActAPSPosn_pct>"
  Bus Selector/3 -> [VINP_LFRawWhlSpeed_kph]  "<VINP_LFRawWhlSpeed_kph>"
  Bus Selector/4 -> [VINP_LRRawWhlSpeed_kph]  "<VINP_LRRawWhlSpeed_kph>"
  Bus Selector/5 -> [VINP_RFRawWhlSpeed_kph]  "<VINP_RFRawWhlSpeed_kph>"
  Bus Selector/6 -> [VINP_RRRawWhlSpeed_kph]  "<VINP_RRRawWhlSpeed_kph>"
  Bus Selector/7 -> [VVMC_LongAcc_Gps]  "<VVMC_LongAcc_Gps>"
  Bus Selector2/1 -> [VTQD_GearActualPosn_enum]  "<VTQD_GearActualPosn_enum>"
  Bus Selector2/2 -> [VTQD_ActWhlSkipSta_enum]  "<VTQD_ActWhlSkipSta_enum>"
  [VTQD_RockModePedTq_Nm] -> VTQD_RockModePedTq_Nm/1
  [VTQD_RockModeTqLim_flg] -> VTQD_RockModeTqLim_flg/1
  MTQD_RockModeDisTime_Y_s/1 -> DelayEnable2/2  "VTQD_RockModeDisTime_s"
  [VTQD_IVIRockModeEn_flg] -> Detect Decrease3/1
  [VTQD_IVIRockModeEn_flg] -> Detect Increase4/1
  AND6/1 -> OR4/1
  [VTQD_VehActSpd_kph] -> Delay13/1
  [task_time_s] -> DelayEnable1/3
  Equal51/1 -> AND2/2
  Delay9/1 -> DelayEnable1/1
  Delay13/1 -> Relational Operator2/1
  OR8/1 -> Detect Decrease2/1
  Constant123/1 -> Equal51/2
  Constant125/1 -> Equal53/2
  [VTQD_IVIRockModeEn_flg] -> Delay7/1
  [VINP_ESCOFFStatus_enum] -> Equal53/1
  [VTQD_RockModeTqLim_flg] -> AND1/1
  Constant124/1 -> Equal52/2
  [VINP_IVIEscapeModeCmd_flg] -> Detect Increase1/1
  Equal52/1 -> AND14/1
  NOT2/1 -> SR_Latch1/2
  Detect Decrease3/1 -> AND14/2
  [VINP_ESCOFFStatus_enum] -> Equal51/1
  [VTQD_GearActualPosn_enum] -> Delay11/1
  Detect Increase1/1 -> AND11/1
  Constant121/1 -> Relational Operator2/2
  AND2/1 -> Detect Increase5/1
  [VPMM_SysPowerMode_enum] -> Relational Operator9/1
  Detect Increase4/1 -> Switch24/2
  Detect Decrease2/1 -> AND1/2
  SR_Latch5/1 -> [VTQD_IVIRockModeEn_flg]  "VTQD_IVIRockModeEn_flg"
  Constant120/1 -> Equal49/2
  Equal50/1 -> Detect Decrease1/1
  [VINP_ESCOFFStatus_enum] -> Equal50/1
  [VTQD_IVIRockModeEn_flg] -> Delay9/1
  Relational Operator9/1 -> AND11/3
  [task_time_s] -> Hold/1
  Detect Increase2/1 -> AND6/1
  Detect Decrease1/1 -> OR4/5
  AND10/1 -> OR4/3
  [VINP_ESCOFFStatus_enum] -> Switch24/1
  Constant127/1 -> Relational Operator9/2
  Constant119/1 -> DelayEnable1/2
  OR4/1 -> SR_Latch5/2  "VTQD_IVIRockModeDis_flg"
  Detect Increase5/1 -> OR5/1
  SR_Latch1/1 -> AND2/1
  Constant128/1 -> Relational Operator10/2
  Delay7/1 -> AND6/2
  [VTQD_FrShaftSpd_rpm] -> Delay14/1
  [VTQD_IVIRockModeEn_flg] -> Delay12/1
  DelayEnable1/1 -> OR4/2
  Switch24/1 -> [VTQD_ESCOFFStaLatch_enum], Delay16/1  "VTQD_ESCOFFStaLatch_enum"
  Constant122/1 -> Equal50/2
  [VTQD_ESCOFFStaLatch_enum] -> Equal52/1
  Detect Increase3/1 -> AND10/2
  Constant129/1 -> Hold/2
  Hold/1 -> [VTQD_RockModeTCSReq_flg]  "VTQD_RockModeTCSReq_flg"
  DelayEnable2/1 -> OR4/4
  Delay12/1 -> DelayEnable2/1
  AND14/1 -> OR5/2
  Delay10/1 -> AND10/1
  Equal49/1 -> Detect Increase3/1
  [VTQD_RrShaftSpd_rpm] -> Delay15/1
  Delay15/1 -> Max2/2
  Max2/1 -> MTQD_RockModeDisTime_Y_s/1
  [VTQD_RockModeTqLim_flg] -> NOT2/1
  Relational Operator2/1 -> AND11/2
  Equal53/1 -> AND14/3
  Relational Operator10/1 -> OR4/6
  Delay14/1 -> Max2/1
  AND1/1 -> SR_Latch1/1
  OR5/1 -> Hold/3
  [VTQD_IVIRockModeEn_flg] -> Delay10/1
  [task_time_s] -> DelayEnable2/3
  [VINP_RrPTCSActive_flg] -> OR8/2
  [VPMM_SysPowerMode_enum] -> Relational Operator10/1
  Delay11/1 -> Equal49/1
  AND11/1 -> SR_Latch5/1
  Delay16/1 -> Switch24/3
  [VINP_IVIEscapeModeCmd_flg] -> Detect Increase2/1
  [VINP_FrPTCSActive_flg] -> OR8/1
  Bus Selector/8 -> [VINP_IVIEscapeModeCmd_flg]  "<VINP_IVIEscapeModeCmd_flg>"
  Bus Selector1/3 -> [VTQD_VehActSpd_kph]  "<VTQD_VehActSpd_kph>"
  Bus Selector/9 -> [VPMM_SysPowerMode_enum]  "<VPMM_SysPowerMode_enum>"
  Bus Selector/1 -> [task_time_s]  "<task_time_s>"
  Bus Selector/10 -> [VINP_ESCOFFStatus_enum]  "<VINP_ESCOFFStatus_enum>"
  Bus Selector/11 -> [VINP_FrPTCSActive_flg]  "<VINP_FrPTCSActive_flg>"
  Bus Selector/12 -> [VINP_RrPTCSActive_flg]  "<VINP_RrPTCSActive_flg>"
  [VTQD_RockModeTCSReq_flg] -> VTQD_RockModeTCSReq_flg/1
  [VTQD_IVIRockModeEn_flg] -> VTQD_IVIRockModeEn_flg/1
  VTQR_FShaftSpdTqLimLow_flg/1 -> [VTQR_FShaftSpdTqLimLow_flg]
  VTQR_FTimerTqLimLow_flg/1 -> [VTQR_FTimerTqLimLow_flg]
  VTQR_RShaftSpdTqLimLow_flg/1 -> [VTQR_RShaftSpdTqLimLow_flg]
  VTQR_RTimerTqLimLow_flg/1 -> [VTQR_RTimerTqLimLow_flg]

== system tqdtqr_rebuild_V3/Input_Convert/Main function/DriverWhlTqDem function/RollingRegenJudge ==
  note: Rolling regen shaft speed
  note: Rolling regen enable condition
  BSCPIn_outputs : Inport
  BSignalConvert_outputs : Inport  Port=2
  VTQD_TqSourceFr_enum : Inport  Port=3
  VTQD_TqSourceRr_enum : Inport  Port=4
  VTQD_CreepEnable_flg : Inport  Port=5
  Bus Selector : BusSelector  OutputSignals=VTQD_LowIdleAccPedal_flg,VINP_VehSpeed_kph
  Bus Selector1 : BusSelector  OutputSignals=VTQD_TqTargetShaftSpd_rpm,VTQD_RollRegenDisable_flg
  Constant : Constant  Value=ENUM_TQSOURCE_CC
  Constant1 : Constant  Value=ENUM_TQSOURCE_ADAS
  Constant2 : Constant  Value=ENUM_TQSOURCE_APS
  Constant3 : Constant  Value=ENUM_TQSOURCE_CC
  Constant4 : Constant  Value=ENUM_TQSOURCE_ADAS
  Constant5 : Constant  Value=ENUM_TQSOURCE_APS
  Delay{,1..5} (6 alike) : Delay  DelayLength=1  InitialCondition=uint8(0)
      settings: AttributesFormatString=%<InitialCondition>
  Detect Increase : simulink/Logic and Bit Operations/Detect Increase  vinit=0.0  OutDataTypeStr=boolean
  Equal{,1..5} (6 alike) : RelationalOperator  Operator===  OutDataTypeStr=boolean  RndMeth=Simplest
  Logical Operator : Logic  Inputs=5  AllPortsSameDT=off  OutDataTypeStr=boolean
  Logical Operator1 : Logic  Operator=NOT  AllPortsSameDT=off  OutDataTypeStr=boolean
  Logical Operator10 : Logic  Operator=OR  AllPortsSameDT=off  OutDataTypeStr=boolean
  Logical Operator11 : Logic  Operator=NOT  AllPortsSameDT=off  OutDataTypeStr=boolean
  Logical Operator12 : Logic  Operator=NOT  AllPortsSameDT=off  OutDataTypeStr=boolean
  Logical Operator5 : Logic  Operator=OR  Inputs=3  AllPortsSameDT=off  OutDataTypeStr=boolean
  Logical Operator9 : Logic  Operator=OR  Inputs=3  AllPortsSameDT=off  OutDataTypeStr=boolean
  Relay : Relay  OnSwitchValue=KTQD_RegenOnSpd_kph  OffSwitchValue=KTQD_RegenOffSpd_kph
      settings: AttributesFormatString=|
      | ON: %<OnSwitchValue>
      | OFF: %<OffSwitchValue>
  Switch2 : Switch  Criteria=u2 ~= 0
      settings: AttributesFormatString=%<Criteria>
  Unit Delay : UnitDelay  InitialCondition=single(0)  SampleTime=-1  HasFrameUpgradeWarning=on
      settings: AttributesFormatString=%<InitialCondition>
  Unit Delay1 : UnitDelay  SampleTime=-1  HasFrameUpgradeWarning=on
  VTQD_RollRegenEnable_flg : Outport
  VTQD_RollingShaftSpd_rpm : Outport  Port=2
  wires:
  Equal5/1 -> Logical Operator9/3
  Equal3/1 -> Logical Operator9/1
  Equal4/1 -> Logical Operator9/2
  Constant4/1 -> Equal4/2
  [VTQD_TqSourceRr_enum] -> Delay4/1
  Constant5/1 -> Equal5/2
  [VTQD_TqSourceRr_enum] -> Delay5/1
  Constant3/1 -> Equal3/2
  [VTQD_TqSourceRr_enum] -> Delay1/1
  Constant2/1 -> Equal2/2
  [VTQD_TqSourceFr_enum] -> Delay2/1
  Constant1/1 -> Equal1/2
  [VTQD_TqSourceFr_enum] -> Delay3/1
  Constant/1 -> Equal/2
  Logical Operator11/1 -> Logical Operator/5
  Logical Operator10/1 -> Logical Operator11/1
  Logical Operator9/1 -> Logical Operator10/2
  Logical Operator5/1 -> Logical Operator10/1
  [VTQD_CreepEnable_flg] -> Unit Delay1/1
  Equal2/1 -> Logical Operator5/3
  Equal1/1 -> Logical Operator5/2
  Equal/1 -> Logical Operator5/1
  VTQD_CreepEnable_flg/1 -> [VTQD_CreepEnable_flg]
  [VTQD_RollRegenDisableReq_flg] -> Logical Operator1/1
  Bus Selector1/2 -> [VTQD_RollRegenDisableReq_flg]  "<VTQD_RollRegenDisable_flg>"
  Unit Delay/1 -> Switch2/3
  Switch2/1 -> VTQD_RollingShaftSpd_rpm/1, Unit Delay/1  "VTQD_RollingShaftSpd_rpm"
  [VTQD_TqTargetShaftSpd_rpm] -> Switch2/1
  Detect Increase/1 -> Switch2/2
  [VTQD_RollRegenEnable_flg] -> Detect Increase/1
  Bus Selector1/1 -> [VTQD_TqTargetShaftSpd_rpm]  "<VTQD_TqTargetShaftSpd_rpm>"
  [VINP_VehSpd_kph] -> Relay/1
  Bus Selector/2 -> [VINP_VehSpd_kph]  "<VINP_VehSpeed_kph>"
  Bus Selector/1 -> [VTQD_LowIdleAccPedal_flg]  "<VTQD_LowIdleAccPedal_flg>"
  Logical Operator/1 -> VTQD_RollRegenEnable_flg/1, [VTQD_RollRegenEnable_flg]  "VTQD_RollRegenEnable_flg"
  Unit Delay1/1 -> Logical Operator12/1
  Relay/1 -> Logical Operator/2
  Logical Operator12/1 -> Logical Operator/4
  Logical Operator1/1 -> Logical Operator/3
  [VTQD_LowIdleAccPedal_flg] -> Logical Operator/1
  [VTQD_TqSourceFr_enum] -> Delay/1
  BSCPIn_outputs/1 -> Bus Selector/1
  BSignalConvert_outputs/1 -> Bus Selector1/1
  Delay/1 -> Equal/1
  VTQD_TqSourceFr_enum/1 -> [VTQD_TqSourceFr_enum]
  VTQD_TqSourceRr_enum/1 -> [VTQD_TqSourceRr_enum]
  Delay3/1 -> Equal1/1
  Delay2/1 -> Equal2/1
  Delay1/1 -> Equal3/1
  Delay4/1 -> Equal4/1
  Delay5/1 -> Equal5/1
